simulink model "Free_Flight"  (R2016a)
settings: configuration reference "AR_Drone_ConfigSet" (kept outside this file)
undefined symbols (not defined in the file or in its folder): accelerometerXyzGains, accelerometerXyzOffsets, DiscIntNeverNeededParam, Drone_StateModeType, fdesignblkfcn, gcbh, gyroXyzOffsets, Mag_Calib_Gain_Vector, Mag_Calib_Offset_Vector
libraries: simulink x7, AR_Drone_Sensors x3, AR_Drone_Actuators x2, vrlib x2, instrumentlib x1
(part 2 of 2)

== system Free_Flight/Vicon data through UDP/Calculate Body Frame Velocities/Lowpass Filter2 ==
  In : Inport
  Generated Filter Block : DiscreteFir  Tag=BlockMethodSubSystem  Coefficients=[0.0010438901225940831 0.00012354088148469351 0.00013070400115602399 0.00013834960280678036 0.00014596894146551005 0.00015403893168281359 0.00016203788292356918 0.00017055350569484217 0.00017907272657582301 0.00018831462117422986 0.00019765090346090652 0.00020784032141500067 0.00021767613324712772 0.00022794168442264817 0.00023659510580732745 0.00024880763191149631 0.00025982277257009573 0.00027040920537772014 0.00028234139711577643 0.00029386124097289601 0.00030624165518130771 0.00031856492905945753 0.00033157294629216011 0.0003445681564084828 0.00035808157890128824 0.00037157915937724819 0.00038570725102277613 0.00040003603069277448 0.0004150893606755414 0.00042970531424921926 0.00044493966348178318 0.00046085727937534454 0.00047660737867372084 0.00049301498023465566 0.00050956455082891157 0.0005265169938793332 0.00054372014428463397 0.00056130805099947521 0.0005792408532847165 0.00059756096394782338 0.0006161512503316352 0.00063502577047820619 0.00065421457556422537 0.0006739226870995439 0.00069396118060180445 0.00071404528982047509 0.0007348193050352688 0.00075568971982121623 0.00077700693244347444 0.00079863279711671017 0.00082062238264760307 0.00084292239903858816 0.00086553173206488181 0.00088844855846355233 0.00091173530528628702 0.00093537667142473268 0.00095932345213913678 0.00098351429226786052 0.0010080262831828227 0.0010330069942687532 0.0010581143509964313 0.0010836336364360136 0.001109463664928924 0.0011355293917327169 0.0011619534649647178 0.0011886280789465049 0.0012156698631213014 0.0012429654101590152 0.0012705580415228951 0.0012983830023958762 0.0013265479795755504 0.001354993647408586 0.0013837340640601783 0.0014126350481840399 0.0014419261003762306 0.0014714130799663582 0.0015011333695863142 0.0015311730914253831 0.0015614041068926483 0.0015919029258883212 0.0016225913209598534 0.0016535206600493311 0.0016846845100252006 0.0017160731807948006 0.0017476400685308582 0.0017793928875518793 0.0018113464482121318 0.0018435274156758802 0.0018758311748156844 0.001908318812522186 0.0019410202594715561 0.0019737934332837949 0.0020067752219371428 0.002039872015752607 0.0020731325612166384 0.0021065119403655846 0.0021399891885268527 0.0021735829551047673 0.0022072955644629215 0.0022411159135527774 0.0022750080964725602 0.0023089674681463935 0.0023430221050463888 0.0023771445752303164 0.0024112712791678433 0.0024455199876448684 0.0024797578031685147 0.0025140351181737065 0.0025483210653412343 0.0025826141369817597 0.0026169333177995069 0.0026512294580176106 0.0026854959299529913 0.0027197299895173649 0.0027539349518122393 0.0027880981426283221 0.0028221849623515875 0.0028562037711923017 0.00289017425063803 0.002924006033889807 0.00295775987972011 0.0029914204082208623 0.0030249432182058887 0.0030583585671591002 0.0030915958463266437 0.0031247114288090599 0.0031576658846565551 0.0031904568769100415 0.0032230561579368704 0.0032554700040130506 0.0032876899050400055 0.0033197046388299609 0.0033514760356486398 0.0033830587602360516 0.0034143897209073628 0.0034454509630193518 0.0034762784604740428 0.0035068197614344736 0.0035371132038200023 0.0035671004556680373 0.003596785990705815 0.0036261729309091544 0.0036552450425178747 0.0036839934327410301 0.0037124021185351544 0.0037404679590860787 0.0037681950789115858 0.0037955321897746325 0.0038225051511365576 0.0038491223019023321 0.0038753262227017014 0.0039011429505233105 0.003926538886960422 0.0039515250460640658 0.0039761051326994666 0.0040002299223065741 0.0040239296135573714 0.004047169367580164 0.0040699648417800646 0.0040922859863476921 0.00411413656626678 0.0041355187713854654 0.0041564202711735047 0.0041767935359899502 0.0041966996825622705 0.0042160831749616951 0.0042349667294033985 0.0042533205776213228 0.0042711382044104528 0.004288437491282584 0.0043051923386315423 0.0043213986168101921 0.0043370622014110875 0.0043521611884634517 0.0043667118550219566 0.0043806727294754735 0.0043940731400972117 0.004406912910723584 0.0044191576567501056 0.0044308100349050574 ...(+4780 chars)]  InputProcessing=Columns as channels (frame based)
  Out : Outport
  wires:
  In/1 -> Generated Filter Block/1
  Generated Filter Block/1 -> Out/1

== system Free_Flight/Flight Controller/Supervisory Flight Controller/Attitude_Control/Rate Control/Desired Rates ==
  b3d : Inport
  R : Inport  Port=2
  Derivative : Derivative
  Desired Rates : MATLAB Function  TreatAsAtomicUnit=on
  Omega_DI_D : MATLAB Function  TreatAsAtomicUnit=on
  Rc : MATLAB Function  TreatAsAtomicUnit=on
  kR : Constant  Value=10
  Omegad : Outport
  eR : Outport  Port=2
  wires:
  b3d/1 -> Rc/1(b3d)
  R/1 -> Rc/2(R)
  Rc/1(Rc) -> Omega_DI_D/1(Rc), Derivative/1
  Derivative/1 -> Omega_DI_D/2(Rc_dot)
  Omega_DI_D/1(Omega_DI_D) -> Desired Rates/1(Omega_DI_D)
  Rc/2(R_tilde) -> Desired Rates/2(R_tilde)
  Rc/3(eR) -> Desired Rates/3(eR), eR/1
  Desired Rates/1(Omegad) -> Omegad/1
  kR/1 -> Desired Rates/4(kR)

== system Free_Flight/Flight Controller/Supervisory Flight Controller/Attitude_Control/Rate Control/L1 Adaptive Control ==
  Omega : Inport
  Omegad : Inport  Port=2
  Adaptation Law : Subsystem
  Control Law : Subsystem
  Predictor : Subsystem
  Scope : Scope
  Scope1 : Scope
  norm_of_omega : MATLAB Function  TreatAsAtomicUnit=on
  u_ad : Outport
  wires:
  Omega/1 -> Predictor/3(Omega)
  Predictor/1(Omega Tilde) -> norm_of_omega/1(omega), Adaptation Law/1(Omega_tilde)
  Adaptation Law/1(sigma_hat) -> Control Law/2(sigma_hat), Predictor/2(sigma_hat)
  norm_of_omega/1(Norm_omega) -> Scope/1
  Omegad/1 -> Control Law/1(Omegad)
  Control Law/1(u_ad) -> Scope1/1, u_ad/1, Predictor/1(u_ad)

== system Free_Flight/Flight Controller/Supervisory Flight Controller/Attitude_Control/Rate Control/Nominal Control ==
  Omega : Inport
  Am : Constant  Value=-50*eye(3)
  J_N : Constant  Value=diag([0.002237568000000,0.002985236000000,0.004803740000000])
  Nominal Control : MATLAB Function  TreatAsAtomicUnit=on
  u_m : Outport
  wires:
  Omega/1 -> Nominal Control/3(Omega)
  Am/1 -> Nominal Control/2(Am)
  J_N/1 -> Nominal Control/1(J_N)
  Nominal Control/1(u_m) -> u_m/1

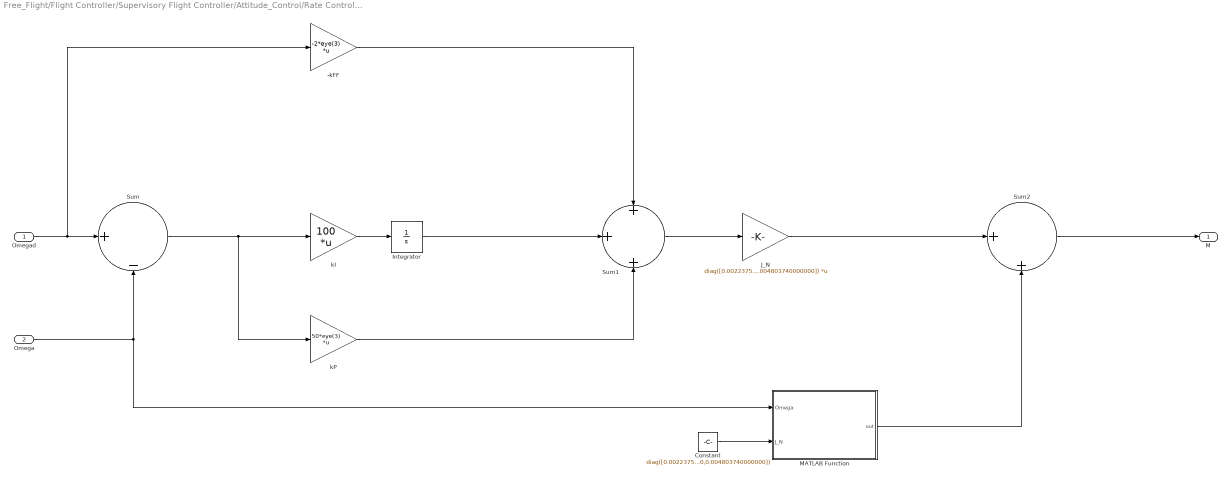
== system Free_Flight/Flight Controller/Supervisory Flight Controller/Attitude_Control/Rate Control/PI for Comparison ==
  Omegad : Inport
  Omega : Inport  Port=2
  -kFF : Gain  Gain=-2*eye(3)  Multiplication=Matrix(K*u)
  Constant : Constant  Value=diag([0.002237568000000,0.002985236000000,0.004803740000000])
  Integrator : Integrator
  J_N : Gain  Gain=diag([0.002237568000000,0.002985236000000,0.004803740000000])  Multiplication=Matrix(K*u)
  MATLAB Function : MATLAB Function  TreatAsAtomicUnit=on
  Sum : Sum  Inputs=|+-
  Sum1 : Sum  Inputs=+|+|+
  Sum2 : Sum  Inputs=|++
  kI : Gain  Gain=100  Multiplication=Matrix(K*u)
  kP : Gain  Gain=50*eye(3)  Multiplication=Matrix(K*u)
  M : Outport
  wires:
  Omegad/1 -> -kFF/1, Sum/1
  Omega/1 -> MATLAB Function/1(Omega), Sum/2
  Sum/1 -> kP/1, kI/1
  kI/1 -> Integrator/1
  -kFF/1 -> Sum1/1
  kP/1 -> Sum1/3
  Sum1/1 -> J_N/1
  J_N/1 -> Sum2/1
  Constant/1 -> MATLAB Function/2(J_N)
  MATLAB Function/1(out) -> Sum2/2
  Sum2/1 -> M/1
  Integrator/1 -> Sum1/2

== system Free_Flight/Navigation System/Kalman Filter/Compute Roll Pitch/Calculate Roll - Pitch ==
  note: http://www.digikey.com/en/articles/techzone/2011/may/using-an-accelerometer-for-inclination-sensing
  Normalized Gravity Vector : Inport
  Gain4 : Gain  Gain=180/pi
  Gain5 : Gain  Gain=-180/pi
  MATLAB Function : MATLAB Function  TreatAsAtomicUnit=on
  RollRaw : Outport
  PitchRaw : Outport  Port=2
  wires:
  Gain5/1 -> PitchRaw/1
  Gain4/1 -> RollRaw/1
  MATLAB Function/2(Pitch) -> Gain5/1  "roll"
  MATLAB Function/1(Roll) -> Gain4/1  "pitch"
  Normalized Gravity Vector/1 -> MATLAB Function/1(Ax_Ay_Az)

== system Free_Flight/Navigation System/Kalman Filter/Compute Roll Pitch/KF_PITCH ==
  GYRO_CTRL_IN : Inport
  PITCH_ACCEL_MEASURE : Inport  Port=2
  Demux : Demux  Outputs=2
  Kalman Tracker : MATLAB Function  TreatAsAtomicUnit=on
  Terminator : Terminator
  Unit Delay : UnitDelay  InitialCondition=eye(2)  SampleTime=-1
  Unit Delay1 : UnitDelay  InitialCondition=[0 0]'  SampleTime=-1
  PITCH_FILTERED : Outport
  wires:
  Demux/2 -> Terminator/1  "B_dot"
  PITCH_ACCEL_MEASURE/1 -> Kalman Tracker/4(measurement_angle)
  Unit Delay/1 -> Kalman Tracker/2(covariance_correction_prev)
  GYRO_CTRL_IN/1 -> Kalman Tracker/3(ctrl_input_gyro)
  Unit Delay1/1 -> Kalman Tracker/1(prev_state)
  Kalman Tracker/1(state_correction) -> Demux/1, Unit Delay1/1
  Demux/1 -> PITCH_FILTERED/1
  Kalman Tracker/2(covariance_correction) -> Unit Delay/1

== system Free_Flight/Navigation System/Kalman Filter/Compute Roll Pitch/KF_ROLL ==
  ROLL_ACCEL_MEASURE : Inport
  GYRO_ROLL_CTRL_IN : Inport  Port=2
  Demux : Demux  Outputs=2
  Kalman Tracker : MATLAB Function  TreatAsAtomicUnit=on
  Terminator : Terminator
  Unit Delay : UnitDelay  InitialCondition=eye(2)  SampleTime=-1
  Unit Delay1 : UnitDelay  InitialCondition=[0 0]'  SampleTime=-1
  ROLL_FILTERED : Outport
  wires:
  Demux/2 -> Terminator/1  "B_dot"
  Demux/1 -> ROLL_FILTERED/1
  ROLL_ACCEL_MEASURE/1 -> Kalman Tracker/4(measurement_angle)
  Unit Delay/1 -> Kalman Tracker/2(covariance_correction_prev)
  GYRO_ROLL_CTRL_IN/1 -> Kalman Tracker/3(ctrl_input_gyro)
  Unit Delay1/1 -> Kalman Tracker/1(prev_state)
  Kalman Tracker/1(state_correction) -> Demux/1, Unit Delay1/1
  Kalman Tracker/2(covariance_correction) -> Unit Delay/1

== system Free_Flight/Navigation System/Kalman Filter/Compute Roll Pitch/Seperate Data ==
  GyroIn : Inport
  Demux1 : Demux  Outputs=[1 1]
  Selector2 : Selector  IndexMode=Zero-based  InputPortWidth=3  IndexOptions=Index vector (dialog)  Indices=[0 1]  OutputSizes=1
  Gyro_Roll_Ctrl : Outport
  Gyro_Pitch_Ctrl : Outport  Port=2
  wires:
  Selector2/1 -> Demux1/1
  Demux1/2 -> Gyro_Pitch_Ctrl/1  "GYRO_Y"
  Demux1/1 -> Gyro_Roll_Ctrl/1  "GYRO_X"
  GyroIn/1 -> Selector2/1

== system Free_Flight/Navigation System/Measurement calibration correction/Accelerometer calibration/Apply calibration parameters ==
  Raw Accelerometer Data : Inport
  Acclerometer Calibration Gains : Constant  Value=accelerometerXyzGains
  Acclerometer Calibration Offsets : Constant  Value=accelerometerXyzOffsets
  Add : Sum  Inputs=+-
  Divide : Product  Inputs=*/
  Invert Axes Definition : Gain  Gain=-1
  Calibrated Accelerometer Data : Outport
  wires:
  Invert Axes Definition/1 -> Calibrated Accelerometer Data/1
  Raw Accelerometer Data/1 -> Add/1
  Acclerometer Calibration Gains/1 -> Divide/2
  Acclerometer Calibration Offsets/1 -> Add/2
  Divide/1 -> Invert Axes Definition/1
  Add/1 -> Divide/1

== system Free_Flight/Navigation System/Measurement calibration correction/Accelerometer calibration/Low pass filter ==
  Offset Accel : Inport
  Add : Sum
  Gain : Gain  Gain=0.8
  Gain1 : Gain  Gain=0.2
  Unit Delay : UnitDelay  SampleTime=-1
  Filtered Accel : Outport
  wires:
  Unit Delay/1 -> Gain/1
  Add/1 -> Unit Delay/1, Filtered Accel/1
  Gain1/1 -> Add/1
  Gain/1 -> Add/2
  Offset Accel/1 -> Gain1/1

== system Free_Flight/Navigation System/Measurement calibration correction/Calibration_Scale_and_Offset/Process Magnetometer ==
  note: magnetometer[ 0 ] = - ( float ) navdata.mx ;
      | magnetometer[ 1 ] = ( float ) navdata.my ;
      | magnetometer[ 2 ] = - ( float ) navdata.mz ;
      | const float Sensitivity[ 3 ] = { 0.0071492608 , 0.0070882491 , 0.0074057781 } ;
      | const float Neutral[ 3 ] = { 118.0 , - 65.0 , 110.0 } ;
  Magnetometer : Inport
  Constant : Constant  Value=[Mag_Calib_Offset_Vector.Gain_X Mag_Calib_Offset_Vector.Gain_Y Mag_Calib_Offset_Vector.Gain_Z]
      settings: AttributesFormatString=%<Value>
  Constant1 : Constant  Value=[Mag_Calib_Gain_Vector.Gain_X Mag_Calib_Gain_Vector.Gain_Y Mag_Calib_Gain_Vector.Gain_Z]
      settings: AttributesFormatString=%<Value>
  Divide : Product  Inputs=/*
  Sum : Sum  Inputs=|+-
  MagVector : Outport
  wires:
  Divide/1 -> MagVector/1
  Constant1/1 -> Divide/1
  Constant/1 -> Sum/2
  Magnetometer/1 -> Sum/1
  Sum/1 -> Divide/2

== system Free_Flight/Navigation System/Measurement calibration correction/Gyro offset/Process Raw Rate Gyro Data ==
  note: const float Sensitivity[ 3 ] = { 0.0609 , 0.0609 , 0.0609 } ;
  Raw Rate Gyro Data : Inport
  Gain : Gain  Gain=[0.0609, 0.0609, 0.0609]  ParamDataTypeStr=double
  Processed Data : Outport
  wires:
  Raw Rate Gyro Data/1 -> Gain/1
  Gain/1 -> Processed Data/1

== system Free_Flight/Flight Controller/Supervisory Flight Controller/Attitude_Control/Rate Control/L1 Adaptive Control/Adaptation Law ==
  Omega_tilde : Inport
  Phi : Constant  Value=4.9938e-05*eye(3)
  Phi1 : Constant  Value=0.9975*eye(3)
  Piecewise Constant Adaptation : MATLAB Function  TreatAsAtomicUnit=on
  sigma_hat : Outport
  wires:
  Omega_tilde/1 -> Piecewise Constant Adaptation/3(Omega_tilde)
  Phi/1 -> Piecewise Constant Adaptation/2(Phi)
  Piecewise Constant Adaptation/1(sigma_hat) -> sigma_hat/1
  Phi1/1 -> Piecewise Constant Adaptation/1(Mat_expm)

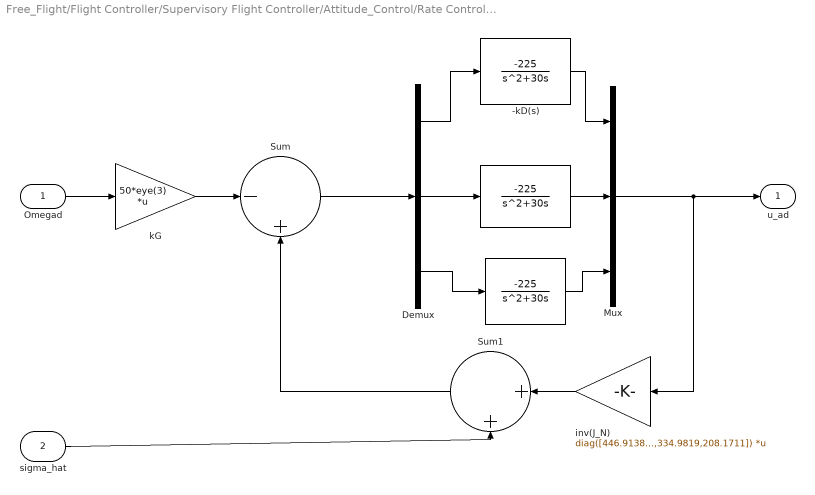
== system Free_Flight/Flight Controller/Supervisory Flight Controller/Attitude_Control/Rate Control/L1 Adaptive Control/Control Law ==
  Omegad : Inport
  sigma_hat : Inport  Port=2
  " " : TransferFcn  Numerator=[0,0,-225]  Denominator=[1,30,0]
  "   " : TransferFcn  Numerator=[0,0,-225]  Denominator=[1,30,0]
  -kD(s) : TransferFcn  Numerator=[0,0,-225]  Denominator=[1,30,0]
  Demux : Demux  Outputs=3
  Mux : Mux  Inputs=3
  Sum : Sum  Inputs=|-+
  Sum1 : Sum  Inputs=|++
  inv(J_N) : Gain  Gain=diag([446.9138,334.9819,208.1711])  Multiplication=Matrix(K*u)
  kG : Gain  Gain=50*eye(3)  Multiplication=Matrix(K*u)
  u_ad : Outport
  wires:
  Omegad/1 -> kG/1
  kG/1 -> Sum/1
  Sum/1 -> Demux/1
  Demux/1 -> -kD(s)/1
  Demux/2 -> " "/1
  Demux/3 -> "   "/1
  -kD(s)/1 -> Mux/1
  " "/1 -> Mux/2
  "   "/1 -> Mux/3
  Mux/1 -> inv(J_N)/1, u_ad/1
  inv(J_N)/1 -> Sum1/1
  sigma_hat/1 -> Sum1/2
  Sum1/1 -> Sum/2

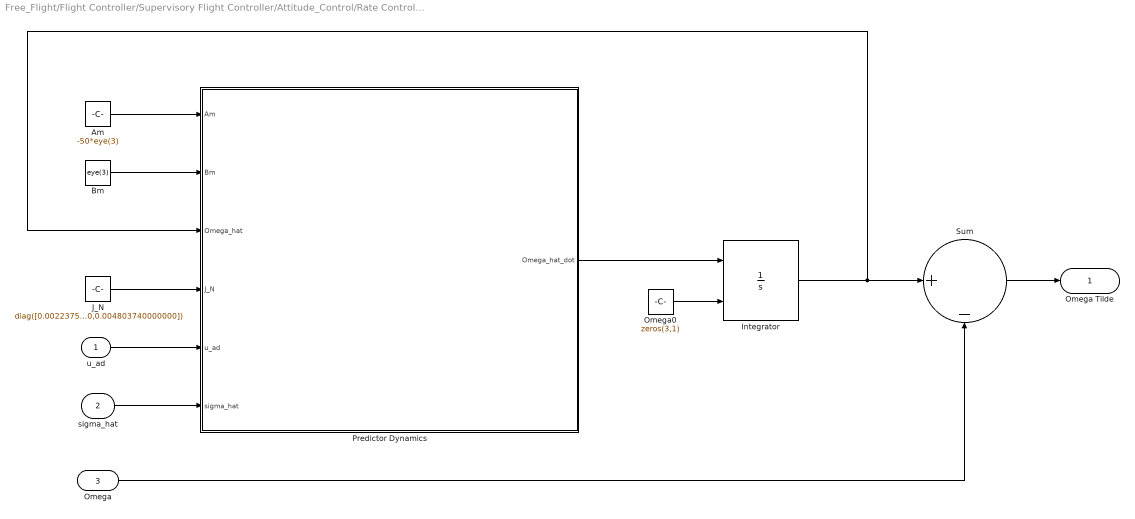
== system Free_Flight/Flight Controller/Supervisory Flight Controller/Attitude_Control/Rate Control/L1 Adaptive Control/Predictor ==
  u_ad : Inport
  sigma_hat : Inport  Port=2
  Omega : Inport  Port=3
  Am : Constant  Value=-50*eye(3)
  Bm : Constant  Value=eye(3)
  Integrator : Integrator  InitialConditionSource=external
  J_N : Constant  Value=diag([0.002237568000000,0.002985236000000,0.004803740000000])
  Omega0 : Constant  Value=zeros(3,1)
  Predictor Dynamics : MATLAB Function  TreatAsAtomicUnit=on
  Sum : Sum  Inputs=|+-
  Omega Tilde : Outport
  wires:
  Am/1 -> Predictor Dynamics/1(Am)
  Bm/1 -> Predictor Dynamics/2(Bm)
  J_N/1 -> Predictor Dynamics/4(J_N)
  sigma_hat/1 -> Predictor Dynamics/6(sigma_hat)
  u_ad/1 -> Predictor Dynamics/5(u_ad)
  Predictor Dynamics/1(Omega_hat_dot) -> Integrator/1
  Omega0/1 -> Integrator/2
  Integrator/1 -> Predictor Dynamics/3(Omega_hat), Sum/1
  Omega/1 -> Sum/2
  Sum/1 -> Omega Tilde/1

== matlab function Free_Flight/Navigation System/Kalman Filter/Compute Roll Pitch/Calculate Roll - Pitch/MATLAB Function ==
  data: Ax_Ay_Az input; Roll output; Pitch output
function [Roll,Pitch] = CalculateAngle(Ax_Ay_Az)
%#codegen
Ax = -Ax_Ay_Az(1);
Ay = -Ax_Ay_Az(2);
Az = Ax_Ay_Az(3);

Pitch = atan( Ax / sqrt( Ay^2 + Az^2));
Roll = atan( Ay / sqrt( Ax^2 + Az^2));

== matlab function Free_Flight/Navigation System/Measurement calibration correction/MATLAB Function ==
  data: Ultrasound_Measure input; UltraSound_Calculation output
function UltraSound_Calculation = removePeak(Ultrasound_Measure)
%#codegen

peakThreshold = 10000;

persistent validHeight
if isempty(validHeight)
    validHeight = 0;
end

if Ultrasound_Measure < peakThreshold
    validHeight = (Ultrasound_Measure - 880) / 26.533;
end

UltraSound_Calculation = validHeight;

== matlab function Free_Flight/Flight Controller/Supervisory Flight Controller/Attitude_Control/Eul2RotM ==
  data: EulAngs input; R output
function R = fcn(EulAngs)
%The Rotation X, Y, and Z from Vicon are exactly the 
%Euler Angles. 
%R is just the rotation matrix from body to inertial frame
%with respect to the geometrical control paper;
R=eul2rotm(EulAngs');
R=R';

== matlab function Free_Flight/Flight Controller/Supervisory Flight Controller/Position_Control/Position Controller ==
  data: x input; fd output; b3d output; v input; R input; Ref input; kx input; kv input; m input; g input
function [fd,b3d] = position_control(x,v,R,Ref,kx,kv,m,g)

xd = Ref(1:3,1); xd_dot = Ref(4:6,1); xd_ddot = Ref(7:9,1);

ex = xd - x; ev = xd_dot - v;

% To help understand: The [0;0;1] is the b3 in body frame.
% R*[0;0;1] is the b3 in inertial frame.

fd = dot((kx*ex + kv*ev +m*g*[0; 0; 1] + m*xd_ddot),R*[0; 0; 1]);

% fd = -(-kx*ex  - kv*ev - m*g*[0; 0; 1]  +m*xd_ddot)'*[0;0;1]/R(3,3); 

b3d = (kx*ex + kv*ev +m*g*[0; 0; 1] + m*xd_ddot)/norm(kx*ex + kv*ev +m*g*[0; 0; 1] + m*xd_ddot);

== matlab function Free_Flight/Flight Controller/Supervisory Flight Controller/Position_Control/  ==
  data: EulAngs input; R output
function R = Eul2RotM1(EulAngs)
%The Rotation Z,Y,X from Vicon are exactly the 
%Euler Angles. 
%R is just the rotation matrix from body to inertial frame
%with respect to the geometrical control paper;
R=eul2rotm(EulAngs');
% This R is from inertial frame to body frame
R=R';
% This R is from body frome to inertial frame

== matlab function Free_Flight/Flight Controller/Supervisory Flight Controller/Drone_State.Controlled_Flight.Altitude_Climb_Step1.E2R/Ref_pva ==
  data: t input; Ref output
function Ref = Reference_trajectories(t)

% Outputs
% xd = desired translational position
% b1d = desired attitude
% So ref is a vetor!!! concluding 9 entries.
% The time is varing.

%% Trajectory 1 (Helix)

% xd = [0.4*t; 0.4*sin(pi*t); 0.6*cos(pi*t)];
% 
% xd_dot = [0.4; 0.4*pi*cos(pi*t); -0.6*pi*sin(pi*t)];
% 
% xd_ddot = [0; -0.4*(pi^2)*sin(pi*t); -0.6*(pi^2)*cos(pi*t)];
% 
% Ref = [xd; xd_dot; xd_ddot];

%% Trajectory 2 (Point Regulation)

% xd = [0; 2; -5];
% 
% xd_dot = [0; 0; 0];
% 
% xd_ddot = [0; 0; 0];
% 
% Ref = [xd; xd_dot; xd_ddot];

%% Trajectory 3 (Circle)

% xd = [10*cos(t); 10*sin(t); 5];
% 
% xd_dot = [-10*sin(t); 10*cos(t); 0];
% 
% xd_ddot = [-10*cos(t); -10*sin(t); 0];
% 
% Ref = [xd; xd_dot; xd_ddot];

%% Trajectory 4 (Heart)

xd = [16*(sin(t))^3; 13*cos(t)-5*cos(2*t)-2*cos(3*t); 0.5];

xd_dot = [48*((sin(t))^2)*cos(t); -13*sin(t)+10*sin(2*t)+6*sin(3*t); 0];

xd_ddot = [96*sin(t)*((cos(t))^2)-48*((sin(t))^2)*cos(t); -13*cos(t)+20*cos(2*t)+18*cos(3*t); 0];

Ref = [xd; xd_dot; xd_ddot];

== matlab function Free_Flight/Flight Controller/Supervisory Flight Controller/Attitude_Control/Rate Control/Desired Rates/Desired Rates ==
  data: Omega_DI_D input; Omegad output; R_tilde input; eR input; kR input
function Omegad = Desired_Rates(Omega_DI_D,R_tilde,eR,kR)

Omegad = R_tilde'*Omega_DI_D - kR*eR;

== matlab function Free_Flight/Flight Controller/Supervisory Flight Controller/Attitude_Control/Rate Control/Desired Rates/Omega_DI_D ==
  data: Rc input; Omega_DI_D output; Rc_dot input
function Omega_DI_D = Omega_DI_D(Rc,Rc_dot)
% Omega_DI_D is the inertial frame's angular velocity in 
% D frame
Omega_DI_D = inverse_skew_symmetric_map(Rc'*Rc_dot);

== matlab function Free_Flight/Flight Controller/Supervisory Flight Controller/Attitude_Control/Rate Control/Desired Rates/Rc ==
  data: b3d input; Rc output; R input; R_tilde output; eR output
function [Rc,R_tilde,eR] = Rc(b3d,R)

%  This b1d could definitely be set randomly. 
%  Since we just want to track the trajectory without requirement for yaw
b1d = (cross(abs(b3d) + ones(3,1),b3d))/norm(cross(abs(b3d) + ones(3,1),b3d));

Rc = [b1d cross(b3d,b1d) b3d];

R_tilde = Rc'*R;

eR = (1/2)*inverse_skew_symmetric_map(R_tilde - R_tilde');

== matlab function Free_Flight/Flight Controller/Supervisory Flight Controller/Attitude_Control/Rate Control/L1 Adaptive Control/norm_of_omega ==
  data: omega input; Norm_omega output
function Norm_omega  = fcn(omega)

Norm_omega = norm(omega);

== matlab function Free_Flight/Flight Controller/Supervisory Flight Controller/Attitude_Control/Rate Control/L1 Adaptive Control/Adaptation Law/Piecewise Constant Adaptation ==
  data: Mat_expm input; sigma_hat output; Phi input; Omega_tilde input
function sigma_hat= piecewise_constant(Mat_expm,Phi,Omega_tilde)

mu = Mat_expm*Omega_tilde;

sigma_hat = -inv(Phi)*mu;

== stateflow chart Free_Flight/Flight Controller/Supervisory Flight Controller ==
  state Fault_Check [parallel]
    settings: executionOrder=3
    state BatteryFault_Check [parallel]
      settings: executionOrder=1
      state BatteryNominal
        en:
        BatteryFault = 0;
        state Nominal
        note: Description:
            | This state will be responsible for the following
            |
            | - Automatically land the drone by forcing it to the land state when voltage is low
            | - Prevent drone from taking off if battery voltage is too low
        state EvaluateVoltageLevel
        state ChangeState
          en:
          BatteryFault = 1;
        EvaluateVoltageLevel -> Fault_Check.BatteryFault_Check.BatteryNominal.Nominal [order 1] : [Measured_Battery_Voltage>=10.1]
        Fault_Check.BatteryFault_Check.BatteryNominal.Nominal -> EvaluateVoltageLevel : [Measured_Battery_Voltage<10.1]
        (default) -> EvaluateVoltageLevel
        EvaluateVoltageLevel -> Fault_Check.BatteryFault_Check.BatteryNominal.ChangeState [order 2] : after(5,sec)
      state BatteryLow
        state ForceLanding
          en:
        (default) -> ForceLanding
      (default) -> BatteryNominal
    state UltraSoundwarning_Check [parallel]
      settings: executionOrder=2
    state SafeOrientation_Check [parallel]
      settings: executionOrder=3
      state UnsafeOrientation
        du:
        MotorArmed =0;
        LandingPhase = 0;
      state WaitForFlight
      state GravityVectorCheck
        en:
        OrientationFault = 0;
        note: Description:
            | This state will be responsible for the following
            |
            | - Automatically land the drone by forcing it to the land state when voltage is low
            | - Prevent drone from taking off if battery voltage is too low
        state Nominal
        state EvaluateGravityVector
        state ChangeState
          en:
          OrientationFault = 1;
        Fault_Check.SafeOrientation_Check.GravityVectorCheck.ChangeState -> Fault_Check.SafeOrientation_Check.GravityVectorCheck.Nominal : [AccelVector_Input<-0.6]
        EvaluateGravityVector -> Fault_Check.SafeOrientation_Check.GravityVectorCheck.Nominal [order 1] : [AccelVector_Input<-0.4]
        Fault_Check.SafeOrientation_Check.GravityVectorCheck.Nominal -> EvaluateGravityVector : [AccelVector_Input>=-0.4]
        (default) -> EvaluateGravityVector
        EvaluateGravityVector -> Fault_Check.SafeOrientation_Check.GravityVectorCheck.ChangeState [order 2] : after(0.01,sec)
      (default) -> WaitForFlight
      GravityVectorCheck -> WaitForFlight : [(hostCmd ==Drone_StateModeType.Landing_Sequence)]
      WaitForFlight -> GravityVectorCheck : [(hostCmd == Drone_StateModeType.Controlled_Flight)]
  state Drone_State [parallel]
    settings: executionOrder=1
    state WaitForHost
      entry:
      reset_offset_calc = 0;
      MotorArmed = 0;
      refStates = zeros(9,1);
      LandingPhase = 0;
      initDone=0;
      note: Description:
          | -This state will wait for the host command to take off
    state Initialize
      entry:
      reset_offset_calc = 0;
      MotorArmed = 0;
      refStates = zeros(9,1);
      LandingPhase = 0;
      initDone=0;
      note: Description:
          | -Upon entry, this block will set the motor to NOT ARMED (turn off integrators in controller, set safety clamp of motors to OFF)
          | -Upon entry, set the refHeight to ZERO
      state Done_Initialization
        entry:
      (default) -> Done_Initialization
    state Controlled_Flight
      entry:
      LandingPhase = 0; refStates =zeros(9,1); MotorArmed =1;
      state Altitude_Climb_Step1
        entry: refStates = E2R();
        state RefStates = E2R [function]
      note: Description:
          | -Upon entry, this block will set the motor to ARMED (enable controller integrator and motor safetey unclamped)
          | -This block will command the AR Drone to fly up to a certain height using the variable refHeight
          | -The output of refHeight should be a function of desired Altitude. The most primitive assignment is to make refHeight = DesiredAltitude, this is comparable to giving the drone a step response. Alternate methods could be giving it a smooth trajectory to follow from the ground to that particular height
          |
          | -Jiaojiao just change it to the calling of a simulink function
      (default) -> Altitude_Climb_Step1
    state Landing_Sequence
      entry:
      note: Description:
          | -Entry into this state will occur if
          | a) Battery drops to around 10.5-10.2 Volts (needs to be experimentally validated)
          | b) Entry condition is met from the user input
          | c) Attitude is out of bounds, ie: the quad rotor has tilted it's pitch to some uncontrollable angle such as 80 degrees
          |
          | Substate goals:
          | -Descend at a controllable rate and land safely
      state Climb_down_1
        entry: LandingPhase=1;
      (default) -> Climb_down_1 : {N=0;}
    state Landing_Terminate
      entry:
      MotorArmed =0;
      LandingPhase = 0;
      %Catch any last state action we need to do here
      note: Description:
          | This state is optional and might not be needed. Up to you if you think having an extra state for the landing phase might be useful.. if not, delete it and consolidate it into previous state
    (default) -> WaitForHost
    Landing_Terminate -> WaitForHost : [sum(MotorCmd)==0]
    WaitForHost -> Initialize : [ (hostCmd == Drone_StateModeType.Controlled_Flight)...
        | && in(Fault_Check.BatteryFault_Check.BatteryNominal.Nominal)...
        | && in (Fault_Check.SafeOrientation_Check.GravityVectorCheck.Nominal)]
    Controlled_Flight -> Landing_Sequence : [(hostCmd == Drone_StateModeType.Landing_Sequence)...
        | ||in(Fault_Check.BatteryFault_Check.BatteryNominal.ChangeState) ...
        | ||in(Fault_Check.SafeOrientation_Check.GravityVectorCheck.ChangeState)]
    Landing_Sequence -> Landing_Terminate : [sum(MotorCmd)==0]
    Done_Initialization -> Controlled_Flight : [after(0.1,sec)]
  state Flight_Controls [parallel]
    settings: executionOrder=2
    state Attitude_Command [parallel]
      entry, during:
      [Attitude_Moment,eR] = Attitude_Control(Euler_Angles,Angular_Velocity,b3d,MotorArmed);
      settings: executionOrder=1
    state Altitude_Command [parallel]
      entry, during:
      [delta_Thrust,b3d] = Position_Control(Trans_XYZ_Feedb,Velo_XYZ_Feedb,refStates,Euler_Angles);
      settings: executionOrder=2
    state MotorMixing_Command [parallel]
      entry, during:
      throttle = NominalThrust+EnableAltitudeCtrl*delta_Thrust;
      MotorCmd = Motor_Mixing(throttle,Attitude_Moment,LandingPhase,MotorArmed);
      settings: executionOrder=3
  state [Moment_controls,eR] = Attitude_Control(EulerAngle_Feedback_Deg,RateGyro_Feedback_Deg,b3d) [function]
  state [b3d,deltaThrottle] = Position_Control(TransXYZ_fb,Velo_XYZ,refStates,Euler_Angles) [function]
  state MotorCommands = Motor_Mixing(throttle,RPYCmd,LandingPhase,Motor_Armed) [function]
  data: RefStates function_output int16; Moment_controls function_output int16 size=3; eR function_output int16 size=3; EulerAngle_Feedback_Deg function_input double size=3; RateGyro_Feedback_Deg function_input double size=3; b3d function_input double size=3; b3d function_output; TransXYZ_fb function_input double size=3; Velo_XYZ function_input double size=1; refStates function_input double size=1; Euler_Angles function_input double size=3; deltaThrottle function_output int16; throttle function_input int16 size=1; RPYCmd function_input int16 size=3; LandingPhase function_input double size=1; MotorCommands function_output; Motor_Armed function_input double size=1; hostCmd input Enum: Drone_StateModeType; UltraSound_Feedback input size=2; initDone local; MotorCmd output size=4; throttle local int16; Euler_Angles input; Angular_Velocity input; AccelVector_Input input; NominalThrust input; EnableAltitudeCtrl input; Drone_StateMode output Enum: Drone_StateModeType; Measured_Battery_Voltage input; Attitude_Thrust local; Altitude_Thrust local; reset_offset_calc local; MotorArmed local; LandingPhase local; N local; BatteryFault local; OrientationFault local; BatteryFault_Mode output Enum: BatteryFault_ModeType; SafeOrientation_Mode output Enum: SafeOrientation_ModeType; refStates output; Trans_XYZ_Feedb input; Velo_XYZ_Feedb input; eR output; b3d local; delta_Thrust local; Attitude_Moment local
  data hostCmd settings: description=|
      | The hostCmd can take the values 0,1 and 2.
      | 
      | 0 - default state when the drone is powered up.
      | 1 - Takeoff
      | 2 - Landing
  data UltraSound_Feedback settings: description=Ultrasound Feedback will contain data on current height (cm) and altitude rate (cm/s)
  data initDone settings: description=A flag to check whether the calibration is done.
  data NominalThrust settings: description=Nominal thrust input (approximately 60% duty cycle)
  data EnableAltitudeCtrl settings: description=A flag to enable the altitude controller
  data refStates settings: description=Desired height at which the drone needs to hover.

== matlab function Free_Flight/Flight Controller/Supervisory Flight Controller/Attitude_Control/Rate Control/L1 Adaptive Control/Predictor/Predictor Dynamics ==
  data: Am input; Omega_hat_dot output; Bm input; Omega_hat input; J_N input; u_ad input; sigma_hat input
function Omega_hat_dot = predictor_dynamics(Am,Bm,Omega_hat,J_N,u_ad,sigma_hat)

Omega_hat_dot = Am*Omega_hat + Bm*(inv(J_N)*u_ad) + sigma_hat;

== matlab function Free_Flight/Flight Controller/Supervisory Flight Controller/Attitude_Control/Rate Control/Nominal Control/Nominal Control ==
  data: J_N input; u_m output; Am input; Omega input
function u_m = nominal_control(J_N,Am,Omega)

u_m = J_N*Am*Omega + cross(Omega,J_N*Omega);

== matlab function Free_Flight/Navigation System/Kalman Filter/Compute Roll Pitch/KF_ROLL/Kalman Tracker ==
  data: prev_state input; covariance_correction_prev input; state_correction output; covariance_correction output; ctrl_input_gyro input; measurement_angle input
function [state_correction, covariance_correction] = fcn(prev_state, covariance_correction_prev, ctrl_input_gyro, measurement_angle)


%-------------------------------
%-------------------------------
%---- Predict Stage ------------
%-------------------------------
%-------------------------------
% pix_value = 5;
Ts = 1/400;
%Process Noise
p_var =0.01;
Q = [p_var^2     0         
      0         p_var^2];

%A matrix
A =  [1   -Ts 
      0   1];

%odutput these values with a unit delay (for algebraic loop), apply initial conditions
state_prediction = A*prev_state + [Ts 0; 0 0]*[ctrl_input_gyro; 0 ];
covariance_prediction = A*covariance_correction_prev*A' + Q;

%-------------------------------
%-------------------------------
%---- Estimate Stage -----------
%-------------------------------
%-------------------------------

    %H matrix
    H = [1 0];

    %Measurement noise from accelerometer angle measurement
    m_var = 0.5;
%     m_var_r = 1;

    R = [m_var^2 ];

    %Measurement Z
    Z = [measurement_angle];

    %Compute Kalman Gain
    Kalman_Gain = covariance_prediction*H'*inv(H*covariance_prediction*H'+R); %2x2 matrix

    %compute state space correction based on measurement
    state_correction = state_prediction + Kalman_Gain*(Z - H*state_prediction); %4x1 vector of states

    %compute covariance correction
    covariance_correction = (eye(2) - Kalman_Gain*H)*covariance_prediction; %2x2 covariance matrix

%     corrected_angle_measure = state_correction(1) - Ts*state_correction(2);
end

== matlab function Free_Flight/Navigation System/Kalman Filter/Compute Roll Pitch/KF_PITCH/Kalman Tracker ==
  data: prev_state input; covariance_correction_prev input; state_correction output; covariance_correction output; ctrl_input_gyro input; measurement_angle input
function [state_correction, covariance_correction] = fcn(prev_state, covariance_correction_prev, ctrl_input_gyro, measurement_angle)


%-------------------------------
%-------------------------------
%---- Predict Stage ------------
%-------------------------------
%-------------------------------
% pix_value = 5;
Ts = 1/400;
%Process Noise
p_var =0.01;
Q = [p_var^2     0         
      0         p_var^2];

%A matrix
A =  [1   -Ts 
      0   1];

%odutput these values with a unit delay (for algebraic loop), apply initial conditions
state_prediction = A*prev_state + [Ts 0; 0 0]*[ctrl_input_gyro; 0 ];
covariance_prediction = A*covariance_correction_prev*A' + Q;

%-------------------------------
%-------------------------------
%---- Estimate Stage -----------
%-------------------------------
%-------------------------------

    %H matrix
    H = [1 0];

    %Measurement noise from accelerometer angle measurement
    m_var = 1;
%     m_var_r = 1;

    R = [m_var^2 ];

    %Measurement Z
    Z = [measurement_angle];

    %Compute Kalman Gain
    Kalman_Gain = covariance_prediction*H'*inv(H*covariance_prediction*H'+R); %2x2 matrix

    %compute state space correction based on measurement
    state_correction = state_prediction + Kalman_Gain*(Z - H*state_prediction); %4x1 vector of states

    %compute covariance correction
    covariance_correction = (eye(2) - Kalman_Gain*H)*covariance_prediction; %2x2 covariance matrix

%     corrected_angle_measure = state_correction(1) - Ts*state_correction(2);
end

== matlab function Free_Flight/Flight Controller/Supervisory Flight Controller/Attitude_Control/Rate Control/PI for Comparison/MATLAB Function ==
  data: Omega input; out output; J_N input
function out = fcn(Omega,J_N)

out = cross(Omega,J_N*Omega);

== matlab function Free_Flight/Navigation System/Kalman Filter/Ultrasound Estimator/Kalman Tracker ==
  data: UltraSoundMeasure input; state_correction output; covariance_correction output; covariance_correction_input input; state_correction_input input
function [state_correction, covariance_correction] = fcn(UltraSoundMeasure, covariance_correction_input,state_correction_input)


%-------------------------------
%-------------------------------
%---- Predict Stage ------------
%-------------------------------
%-------------------------------

%our states:
%  [Wx Wy Wz Bx By Bz   ]
%

p_var = 1e-2;
Ts = 1/400;
%Process Noise

Q = [p_var^2     0     
      0         p_var^2 ];

%A matrix
A =  [1   Ts    
      0   1];

%odutput these values with a unit delay (for algebraic loop), apply initial conditions
state_prediction = A*state_correction_input;
covariance_prediction_ = A*covariance_correction_input*A' + Q;

%-------------------------------
%-------------------------------
%---- Estimate Stage -----------
%-------------------------------
%-------------------------------
    %H matrix
    H = [1 0];

    %Measurement noise
    m_var = 1;
%     m_var_r = 1;

    R = [m_var^2];

    %Measurement Z
    Z = UltraSoundMeasure;

    %Compute Kalman Gain
    Kalman_Gain = covariance_prediction_*H'*inv(H*covariance_prediction_*H'+R); %2x2 matrix

    %compute state space correction based on measurement
    state_correction = state_prediction + Kalman_Gain*(Z - H*state_prediction); %2x1 vector of states

    %compute covariance correction
    covariance_correction = (eye(2) - Kalman_Gain*H)*covariance_prediction_; %2x2 covariance matrix

end

== matlab function Free_Flight/Flight Controller/Supervisory Flight Controller/Motor_Mixing/RampDownInSpeed1 ==
  data: Cmd input; motorCmd output; stopCmd input
function motorCmd = fcn(Cmd,stopCmd)
%#codegen
persistent tempCmd;
if(isempty(tempCmd))
    tempCmd = ([0;0;0;0]);
end
if(stopCmd)
    tempCmd = tempCmd + ([1;1;1;1]*15/400);
    motorCmd = Cmd - tempCmd;
    
else
    tempCmd = ([0;0;0;0]);
    motorCmd = Cmd;
end

% if (motorCmd(1) <=0)
%         motorCmd = ([0;0;0;0]);
% end

%apply lower bounding
for i=1:4
    
if motorCmd(i)<0
    motorCmd(i) = 0;
end

end

== matlab function Free_Flight/Vicon data through UDP/MATLAB Function ==
  data: phi input; roll output
function roll = f(phi)
roll = phi;
phi = phi*(180/pi);

%Vicon assumes zero roll as the drone is upside down.
%To remedy this, the values are rotated so that 0 is right-side
%up and positive roll is to the right. 
%The value of 90 is just an arbitrary value as Vicon seems to 
%output values between either -160 to -190, or 160-190.

if (phi >= 90)
    roll = phi - 180;
    roll = roll*(pi/180);
end
if (phi <= -90)
    roll = 180 - (phi*-1);
    roll = roll*(pi/180);
end
